simulink model "Copy_of_can_simple_block"  (Simulink 8.8)
settings: Solver=FixedStepDiscrete  StartTime=0.0  StopTime=1000  FixedStep=0.2  RelTol=1e-3  EnableMultiTasking=on
undefined symbols (not defined in the file or in its folder): A, A14, B, B13, B7, C, CS0, D, D4, F3, F4, G3, G4, H3, H4, K17, K4, L3, N16, N3, P3, PD4, PD5, PD6, R10, R14, SCK, SIN, SOUT, T14
libraries: rappid_564xl_ec_toolbox x16
settings Model: Creator=RMuradov  LastModifiedBy=User
settings DataIOCC: ExternalInput=off  InitialState=off  SaveOutput=off  SignalLogging=off  SaveTime=off
settings OptimizationCC: DefaultParameterBehavior=Inlined  ExpressionDepthLimit=2147483647  LifeSpan=1
settings DebuggingCC: SolverPrmCheckMsg=warning  InheritedTsInSrcMsg=none  SingleTaskRateTransMsg=error  UnconnectedInputMsg=error  UnconnectedOutputMsg=error  UnconnectedLineMsg=error  UnknownTsInhSupMsg=error
settings HardwareCC: ProdLargestAtomicInteger=Long  ProdLargestAtomicFloat=Double  ProdIntDivRoundTo=Zero  ProdEndianess=BigEndian  ProdHWDeviceType=Freescale->32-bit PowerPC
settings SFSimCC: SimCustomInitializer=init_PEC15_table();
settings SFSimCC: SimCustomHeaderCode=|
  | #include "doubleIt.h"
  | #include "PEC15.h"
settings SFSimCC: SimUserSources=|
  | doubleIt.c
  | PEC15.c
settings RTWCC: SystemTargetFile=rappid564xl.tlc  MakeCommand=rappid_564xl_make_rtw  TemplateMakefile=rappid_564xl_default_tmf  PostCodeGenCommand=rappid_analyzegencode(buildInfo)  Description=RAppID Toolbox MPC564xL Code Generation Target (rappid)  TLCAssert=on
settings CodeAppCC: IgnoreCustomStorageClasses=off  CustomSymbolStrType=$N$R$M  InternalIdentifier=Classic
settings STFCustomTargetCC: ModelReferenceCompliant=off  CombineOutputUpdateFcns=on  SuppressErrorStatus=on  ERTCustomFileBanners=on  SupportContinuousTime=off  SupportNonInlinedSFcns=off  RemoveResetFunc=on  MATLABClassNameForMDSCustomization=Simulink.SoftwareTarget.ERTCustomization  GRTInterface=off  SystemTargetFile=rappid564xl.tlc
settings ERTTargetCC: MultiwordLength=2048  ModelReferenceCompliant=off  ParMdlRefBuildCompliant=off  CompOptLevelCompliant=off  ConcurrentExecutionCompliant=off  SuppressErrorStatus=on  ERTFirstTimeCompliant=off  ModelStepFunctionPrototypeControlCompliant=off  CPPClassGenCompliant=off  UseToolchainInfoCompliant=off  ExtModeMexFile=noextcomm  InlinedParameterPlacement=NonHierarchical  ERTCustomFileTemplate=example_file_process.tlc  ConvertIfToSwitch=off  SuppressUnreachableDefaultCases=off

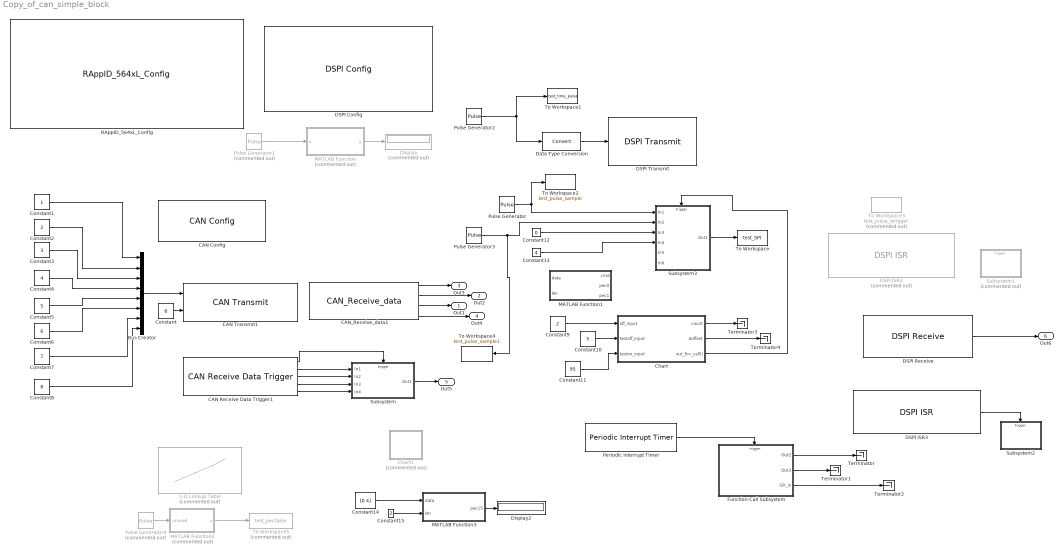
== system Copy_of_can_simple_block ==
  1-D Lookup Table : Lookup_n-D  Commented=on  NumberOfTableDimensions=1  BreakpointsForDimension1=[1:256]  Table="[0\t50585\t52907\t2866\t55503\t7510\t5732\t54269\t62471\t12702\t15020\t65333\t11464\t59729\t57955\t10234\t44439\t26638\t25404\t42661\t30040\t45249\t48115\t32362\t22928\t39945\t38715\t21154\t33119\t17606\t20468\t35437\t23342\t40631\t38277\t20508\t33761\t18040\t19786\t35027\t44841\t27312\t24962\t42011\t30694\t45695\t47437\t31956\t63161\t13088\t14354\t64907\t11894\t60399\t57565\t9540\t702\t50983\t52245\t2444\t55921\t8168\t5338\t53571\t62405\t13916\t15726\t63735\t11018\t61075\t58785\t8248\t1986\t49755\t51561\t3312\t57101\t6804\t4518\t54335\t24146\t39883\t37113\t21856\t34461\t17156\t18486\t36271\t43605\t28620\t25854\t41319\t29338\t46851\t48177\t31144\t43243\t28018\t26176\t41945\t28708\t46525\t48783\t31510\t23788\t39285\t37447\t22494\t33827\t16826\t19080\t36625\t1404\t49381\t52183\t3662\t56755\t6186\t4888\t54913\t61819\t13538\t16336\t64073\t10676\t60461\t59167\t8838\t41491\t26506\t27832\t43297\t31452\t48965\t46199\t29166\t22036\t37773\t39103\t23846\t36571\t19266\t16496\t34281\t3972\t51741\t49455\t1206\t55115\t4818\t6624\t56441\t64387\t15898\t13608\t61617\t9036\t59093\t60903\t10366\t63805\t15524\t14230\t61967\t8690\t58475\t61273\t10944\t3386\t51363\t50065\t1544\t54773\t4204\t7006\t57031\t21674\t37171\t39425\t24472\t35941\t18940\t17102\t34647\t41133\t25908\t28166\t43935\t30818\t48635\t46793\t29520\t20950\t37967\t40829\t23268\t35097\t19584\t18354\t33323\t42449\t24648\t27514\t44771\t32030\t47239\t46005\t30252\t64577\t14808\t13034\t63347\t9358\t57623\t59941\t12220\t2118\t52703\t50925\t884\t53385\t5392\t7714\t56251\t2808\t53089\t50259\t458\t53815\t6062\t7324\t55557\t65279\t15206\t12372\t62925\t9776\t58281\t59547\t11522\t42863\t25334\t27076\t44125\t32672\t47673\t45323\t29842\t21352\t38641\t40387\t22618\t35751\t20030\t17676\t32917]"  InternalRulePriority=Speed  RndMeth=Simplest  InputSameDT=on
  Bus Creator : BusCreator  Inputs=8
  CAN Config : rappid_564xl_ec_toolbox/MPC564xL/Communication Blocks/CAN Config  Priority=1  can_unit=A  can_unit_v2=0  can_idam=A - One full ID (standard or extended) per filter element.  can_srx_dis=1 - Self reception disabled  can_presdiv=4  can_rjw=3  can_pseg1=3  can_pseg2=3  can_clk_src=0 - The CAN engine clock source is the oscillator clock  can_lpb=0 - Loop Back disabled  can_smp=1 - Three samples are used to determine the value of the received bit  can_boff_rec=0 - Automatic recovering from Bus Off state enabled  can_tsyn=0 - Timer Sync feature disabled  can_lbuf=0 - Buffer with highest priority is transmitted first  can_lom=0 - Listen Only Mode is deactivated  can_propseg=6
  CAN Receive Data Trigger1 : rappid_564xl_ec_toolbox/MPC564xL/Communication Blocks/CAN Receive Data Trigger  can_unit=A  can_unit_v2=0  can_buffer=5  can_id=1021  can_isr_prio=14
  CAN Transmit1 : rappid_564xl_ec_toolbox/MPC564xL/Communication Blocks/CAN Transmit  can_unit=A  can_unit_v2=0  can_buffer=14  can_id=1020
  CAN_Receive_data1 : rappid_564xl_ec_toolbox/MPC564xL/Communication Blocks/CAN_Receive_data  can_unit=A  can_unit_v2=0  can_buffer=7  can_id=1010
  Chart : Stateflow chart  TreatAsAtomicUnit=on
  Chart1 : Stateflow chart  Commented=on  TreatAsAtomicUnit=on
  Constant : Constant  Value=8  OutDataTypeStr=uint8
  Constant1 : Constant  OutDataTypeStr=uint8
  Constant10 : Constant  Value=5
  Constant11 : Constant  Value=95
  Constant12 : Constant  Value=0  OutDataTypeStr=Inherit: Inherit via back propagation
  Constant13 : Constant  Value=4  OutDataTypeStr=Inherit: Inherit via back propagation
  Constant14 : Constant  Value=[0 4]  VectorParams1D=off  OutDataTypeStr=uint8
  Constant15 : Constant  Value=2  OutDataTypeStr=Inherit: Inherit via back propagation
  Constant2 : Constant  Value=2  OutDataTypeStr=uint8
  Constant3 : Constant  Value=3  OutDataTypeStr=uint8
  Constant4 : Constant  Value=4  OutDataTypeStr=uint8
  Constant5 : Constant  Value=5  OutDataTypeStr=uint8
  Constant6 : Constant  Value=6  OutDataTypeStr=uint8
  Constant7 : Constant  Value=7  OutDataTypeStr=uint8
  Constant8 : Constant  Value=8  OutDataTypeStr=uint8
  Constant9 : Constant  Value=2
  DSPI Config : rappid_564xl_ec_toolbox/MPC564xL/Communication Blocks/DSPI Config  Priority=1  dspi_Num=1  dspi_Mode=Master  dspi_MTFE=off  dspi_CONT_SCKE=off  dspi_PCSSE=off  dspi_ROOE=off  dspi_DIS_TXF=Enable  dspi_DIS_RXF_v2=Enable  dspi_SMPL_PT=DSPI samples SIN at driving SCK edge  dspi_FMSZ=16  dspi_CPOL=Low  dspi_CPHA=Data is captured on the leading edge of SCK and changed on the following edge  dspi_LSBFE=MSB first  dspi_DBR=off  dspi_PCSSCK=1  dspi_PASC=1  dspi_PDT=5  dspi_PBR=5  dspi_CSSCK=256  dspi_ASC=256  dspi_DT=8  dspi_BR=128  dspi_PCSIS0=High  dspi_PCSIS1=High  dspi_PCSIS2=High  dspi_PCSIS3=High  dspi_PCSIS4=High  dspi_PCSIS5=High  dspi_PCSIS6=High  dspi_PCSIS7=High  dspi_DIS_RXF=Oops
  DSPI ISR2 : rappid_564xl_ec_toolbox/MPC564xL/Communication Blocks/DSPI ISR  Commented=on  dspi_Num=1  dspi_isr_name=TCF - Transfer Complete  dspi_isrPrio=14  dspi_isr_tfuf=off  dspi_isr_rfof=on
  DSPI ISR3 : rappid_564xl_ec_toolbox/MPC564xL/Communication Blocks/DSPI ISR  dspi_Num=1  dspi_isr_name=EOQF - End of Queue  dspi_isrPrio=14  dspi_isr_tfuf=off  dspi_isr_rfof=on
  DSPI Receive : rappid_564xl_ec_toolbox/MPC564xL/Communication Blocks/DSPI Receive  dspi_Num=1
  DSPI Transmit : rappid_564xl_ec_toolbox/MPC564xL/Communication Blocks/DSPI Transmit  Priority=2  dspi_Num=1  dspi_CONT=off  dspi_PUSHR_PE=off  dspi_PUSHR_PP=off  dspi_PCS_0=36 : C[4] : [11] : [H3] : CS0  dspi_PCS_1=5 : A[5] : [14] : [H4] : CS0  dspi_PCS_2=3 : A[3] : [92] : [K17] : CS0  dspi_PCS_slave_0=36 : C[4] : [11] : [H3] : CS0  dspi_PCS_slave_1=5 : A[5] : [14] : [H4] : CS0  dspi_PCS_slave_2=3 : A[3] : [92] : [K17] : CS0  dspi_SIN_0=39 : C[7] : [15] : [K4] : SIN  dspi_SIN_1=8 : A[8] : [12] : [F4]  dspi_SIN_2=2 : A[2] : [84] : [N16] : SIN  dspi_SCK_0=37 : C[5] : [13] : [G3] : SCK  dspi_SCK_1=6 : A[6] : [2] : [G4] : SCK  dspi_SCK_2=0 : A[0] : [73] : [T14] : SCK  dspi_SOUT_0=38 : C[6] : [142] : [D4] : SOUT  dspi_SOUT_1=7 : A[7] : [10] : [F3] : SOUT  dspi_SOUT_2=1 : A[1] : [74] : [R14] : SOUT  dspi_Strobe=None  dspi_eoq=off  dspi_pcsx=Assert
  Data Type Conversion : DataTypeConversion  Priority=1
  Display : Display  Commented=on
  Display2 : Display
  Function-Call Subsystem : Subsystem  TreatAsAtomicUnit=on
      settings: RTWSystemCode=Nonreusable function
  MATLAB Function : MATLAB Function  Commented=on  TreatAsAtomicUnit=on
  MATLAB Function1 : MATLAB Function  TreatAsAtomicUnit=on
  MATLAB Function2 : MATLAB Function  Commented=on  TreatAsAtomicUnit=on
  MATLAB Function3 : MATLAB Function  TreatAsAtomicUnit=on
  Periodic Interrupt Timer : rappid_564xl_ec_toolbox/MPC564xL/General Purpose Blocks/Periodic Interrupt Timer  pit_chan=1  pit_timeout=200  int_priority=12  pit_timeout_val=23999999
  Pulse Generator : DiscretePulseGenerator  Period=100  PhaseDelay=3
  Pulse Generator1 : DiscretePulseGenerator  Commented=on  Amplitude=2  Period=100  PulseWidth=2
  Pulse Generator2 : DiscretePulseGenerator  Period=100
  Pulse Generator3 : DiscretePulseGenerator  Period=100  PhaseDelay=15
  Pulse Generator4 : DiscretePulseGenerator  Commented=on  Amplitude=2  Period=100  PulseWidth=2
  RAppID_564xL_Config : rappid_564xl_ec_toolbox/MPC564xL/RAppID_564xL_Config  SystemClock=120  XTAL=40  MC_clock_60=12  MC_clock_80=16  MC_clock_120=10  SWG_clock_60=20  SWG_clock_80=13.334  SWG_clock_120=20  Compiler=CodeWarrior  MemTarget=RAM  Part=MPC5643L  Package=144 LQFP  global_int_priority=11  base_tick_priority=12  sys_task_supress=off  exception_handlers=off  stored_mdl_name=can_simple_block__  freemaster_interface=Oops  freemaster_rx_pin="LINFlex_0 Rx Pin 116 : \"PB[3]\""  freemaster_tx_pin="LINFlex_0 Tx Pin 114 : \"PB[2]\""  freemaster_interface_1=None  freemaster_enable=off  freemaster_rate=57600  freemaster_tx0_pin=18 : B[2] : 114 : A14  freemaster_rx0_pin=19 : B[3] : 116 : B13  freemaster_tx1_pin=57 : D[9] : 26 : L3  freemaster_rx1_pin=29 : B[13] : 60 : R10  freemaster_can_channel=1CH  freemater_can_speed=500K  freemaster_can_msgig=0x7AA  ccp_interface=None  ccp_enable=off  ccp_can_channel=CH1 (MB 0 - 1)  ccp_can_speed=500K  ccp_can_cro_id=256  ccp_can_dto_id=257  ccp_dev_id=RappID  ccp_dev_addr=0  ccp_odt=3  ccp_daq=3  pil_enable=off  pil_bam=off  comport=1  pil_rate=57600  bam_password_def=on  bam_password=0xFEEDFACECAFEBEEF  bam_sa_cs=off  bam_start_address=0x0  bam_code_size=0x7000  cons_dspi=on  cons_can=on  cons_adc=on  cons_pwm=on  cons_ctu=on  cons_swg=on  cons_eTimer=on  cons_fm=on
  Subsystem : Subsystem
      settings: RTWSystemCode=Nonreusable function
  Subsystem1 : Subsystem  Commented=on
      settings: RTWSystemCode=Nonreusable function
  Subsystem2 : Subsystem
      settings: RTWSystemCode=Nonreusable function
  Subsystem3 : Subsystem
      settings: RTWSystemCode=Nonreusable function
  Terminator{,1..4} (5 alike) : Terminator
  To Workspace : ToWorkspace  VariableName=test_SPI  SaveFormat=Timeseries  SampleTime=-1
  To Workspace1 : ToWorkspace  VariableName=test_time_pulse  SaveFormat=Timeseries  SampleTime=-1
  To Workspace2 : ToWorkspace  VariableName=test_pulse_sample  SaveFormat=Timeseries  SampleTime=-1
  To Workspace3 : ToWorkspace  Commented=on  VariableName=test_pulse_strigger  SaveFormat=Timeseries  SampleTime=-1
  To Workspace4 : ToWorkspace  VariableName=test_pulse_sample1  SaveFormat=Timeseries  SampleTime=-1
  To Workspace5 : ToWorkspace  Commented=on  VariableName=test_pectable  SampleTime=-1
      settings: Save2DSignal=2-D array (concatenate along first dimension)
  Out1 : Outport
  Out2 : Outport  Port=2
  Out3 : Outport  Port=3
  Out4 : Outport  Port=4
  Out5 : Outport  Port=5
  Out6 : Outport  Port=6
  wires:
  Bus Creator/1 -> CAN Transmit1/1
  Constant1/1 -> Bus Creator/1
  Constant2/1 -> Bus Creator/2
  Constant3/1 -> Bus Creator/3
  Constant4/1 -> Bus Creator/4
  Constant5/1 -> Bus Creator/5
  Constant6/1 -> Bus Creator/6
  Constant8/1 -> Bus Creator/8
  Constant7/1 -> Bus Creator/7
  CAN_Receive_data1/4 -> Out4/1
  CAN_Receive_data1/3 -> Out1/1
  CAN_Receive_data1/2 -> Out2/1
  CAN_Receive_data1/1 -> Out3/1
  Constant/1 -> CAN Transmit1/2
  CAN Receive Data Trigger1/3 -> Subsystem/2(In2)
  CAN Receive Data Trigger1/4 -> Subsystem/3(In3)
  CAN Receive Data Trigger1/5 -> Subsystem/4(In4)
  CAN Receive Data Trigger1/2 -> Subsystem/1(In1)
  CAN Receive Data Trigger1/1 -> Subsystem/Trigger
  Subsystem/1(Out1) -> Out5/1
  DSPI Receive/1 -> Out6/1
  DSPI ISR3/1 -> Subsystem2/Trigger
  Data Type Conversion/1 -> DSPI Transmit/1
  Periodic Interrupt Timer/1 -> Function-Call Subsystem/Trigger
  Function-Call Subsystem/1(Out2) -> Terminator/1
  Function-Call Subsystem/2(Out3) -> Terminator1/1
  Function-Call Subsystem/3(SPI_in) -> Terminator2/1
  Pulse Generator/1 -> Subsystem3/1(In1), To Workspace2/1
  Subsystem3/1(Out1) -> To Workspace/1
  Pulse Generator1/1 -> MATLAB Function/1(u)
  MATLAB Function/1(y) -> Display/1
  Pulse Generator2/1 -> Data Type Conversion/1, To Workspace1/1
  Chart/1(count) -> Terminator3/1
  Chart/2(" Aoffset") -> Terminator4/1
  Chart/3(out_fcn_call()) -> Subsystem3/Trigger
  Pulse Generator3/1 -> Subsystem3/2(In2), To Workspace4/1
  Constant9/1 -> Chart/1(off_input)
  Constant10/1 -> Chart/2(testoff_input)
  Constant11/1 -> Chart/3(teston_input)
  MATLAB Function2/1(y) -> To Workspace5/1
  Pulse Generator4/1 -> MATLAB Function2/1(unused)
  Constant14/1 -> MATLAB Function3/1(data)
  Constant15/1 -> MATLAB Function3/2(len)
  MATLAB Function3/1(pec15) -> Display2/1
  Constant12/1 -> Subsystem3/3(In3)
  Constant13/1 -> Subsystem3/4(In4)

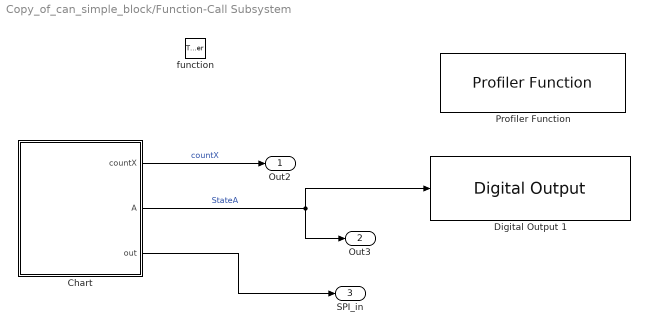
== system Copy_of_can_simple_block/Function-Call Subsystem ==
  function : TriggerPort  TriggerType=function-call  VariantControl=Variant
  Chart : Stateflow chart  TreatAsAtomicUnit=on
  Digital Output 1 : rappid_564xl_ec_toolbox/MPC564xL/General Purpose Blocks/Digital Output   gpio_outputs="52  : PD4  : [ 129 ] : [ B7 ]"  pinNum=[ 129 ]  pcrNum=52
  "Profiler Function " : rappid_564xl_ec_toolbox/MPC564xL/Utility Blocks/Profiler Function   profile_indx=0
  Out2 : Outport
  Out3 : Outport  Port=2
  SPI_in : Outport  Port=3
  wires:
  Chart/1(countX) -> Out2/1  "countX"
  Chart/2(" A") -> Out3/1, Digital Output 1/1  "StateA"
  Chart/3(out) -> SPI_in/1

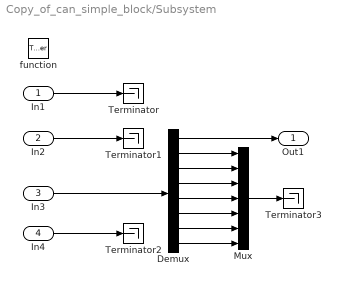
== system Copy_of_can_simple_block/Subsystem ==
  In1 : Inport
  In2 : Inport  Port=2
  In3 : Inport  Port=3
  In4 : Inport  Port=4
  function : TriggerPort  TriggerType=function-call  VariantControl=Variant
  Demux : Demux  Outputs=8
  Mux : Mux  Inputs=7
  Terminator{,1..3} (4 alike) : Terminator
  Out1 : Outport
  wires:
  In1/1 -> Terminator/1
  In2/1 -> Terminator1/1
  In4/1 -> Terminator2/1
  In3/1 -> Demux/1
  Demux/8 -> Mux/7
  Demux/7 -> Mux/6
  Demux/6 -> Mux/5
  Demux/5 -> Mux/4
  Demux/4 -> Mux/3
  Demux/3 -> Mux/2
  Demux/2 -> Mux/1
  Mux/1 -> Terminator3/1
  Demux/1 -> Out1/1

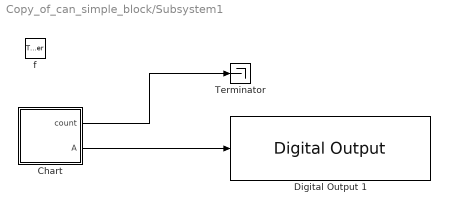
== system Copy_of_can_simple_block/Subsystem1 ==
  f : TriggerPort  TriggerType=function-call  VariantControl=Variant
  Chart : Stateflow chart  TreatAsAtomicUnit=on
  Digital Output 1 : rappid_564xl_ec_toolbox/MPC564xL/General Purpose Blocks/Digital Output   gpio_outputs="53  : PD5  : [ 33 ] : [ N3 ]"  pinNum=[ 33 ]  pcrNum=53
  Terminator : Terminator
  wires:
  Chart/1(count) -> Terminator/1
  Chart/2(" A") -> Digital Output 1/1

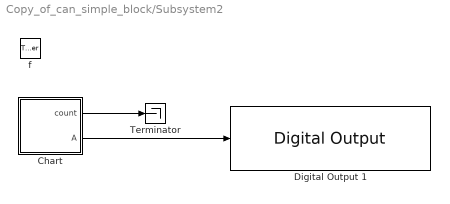
== system Copy_of_can_simple_block/Subsystem2 ==
  f : TriggerPort  TriggerType=function-call  VariantControl=Variant
  Chart : Stateflow chart  TreatAsAtomicUnit=on
  Digital Output 1 : rappid_564xl_ec_toolbox/MPC564xL/General Purpose Blocks/Digital Output   gpio_outputs="54  : PD6  : [ 34 ] : [ P3 ]"  pinNum=[ 34 ]  pcrNum=54
  Terminator : Terminator
  wires:
  Chart/1(count) -> Terminator/1
  Chart/2(" A") -> Digital Output 1/1

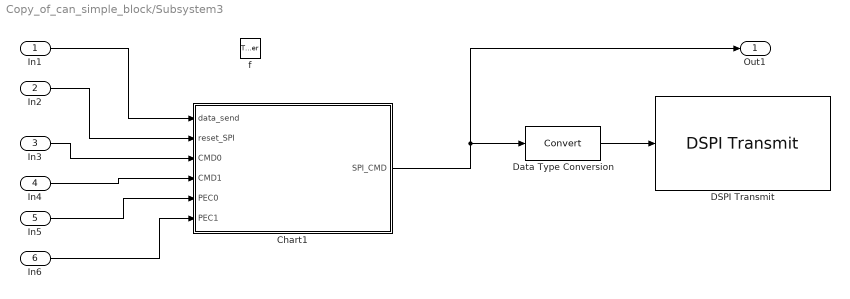
== system Copy_of_can_simple_block/Subsystem3 ==
  In1 : Inport
  In2 : Inport  Port=2
  In3 : Inport  Port=3
  In4 : Inport  Port=4
  In5 : Inport  Port=5
  In6 : Inport  Port=6
  f : TriggerPort  TriggerType=function-call  VariantControl=Variant
  Chart1 : Stateflow chart  TreatAsAtomicUnit=on
  DSPI Transmit : rappid_564xl_ec_toolbox/MPC564xL/Communication Blocks/DSPI Transmit  Priority=2  dspi_Num=1  dspi_CONT=off  dspi_PUSHR_PE=off  dspi_PUSHR_PP=off  dspi_PCS_0=36 : C[4] : [11] : [H3] : CS0  dspi_PCS_1=5 : A[5] : [14] : [H4] : CS0  dspi_PCS_2=3 : A[3] : [92] : [K17] : CS0  dspi_PCS_slave_0=36 : C[4] : [11] : [H3] : CS0  dspi_PCS_slave_1=5 : A[5] : [14] : [H4] : CS0  dspi_PCS_slave_2=3 : A[3] : [92] : [K17] : CS0  dspi_SIN_0=39 : C[7] : [15] : [K4] : SIN  dspi_SIN_1=8 : A[8] : [12] : [F4]  dspi_SIN_2=2 : A[2] : [84] : [N16] : SIN  dspi_SCK_0=37 : C[5] : [13] : [G3] : SCK  dspi_SCK_1=6 : A[6] : [2] : [G4] : SCK  dspi_SCK_2=0 : A[0] : [73] : [T14] : SCK  dspi_SOUT_0=38 : C[6] : [142] : [D4] : SOUT  dspi_SOUT_1=7 : A[7] : [10] : [F3] : SOUT  dspi_SOUT_2=1 : A[1] : [74] : [R14] : SOUT  dspi_Strobe=None  dspi_eoq=off  dspi_pcsx=Assert
  Data Type Conversion : DataTypeConversion  Priority=1
  Out1 : Outport
  wires:
  Chart1/1(SPI_CMD) -> Data Type Conversion/1, Out1/1
  In1/1 -> Chart1/1(data_send)
  Data Type Conversion/1 -> DSPI Transmit/1
  In2/1 -> Chart1/2(reset_SPI)
  In3/1 -> Chart1/3(CMD0)
  In4/1 -> Chart1/4(CMD1)
  In5/1 -> Chart1/5(PEC0)
  In6/1 -> Chart1/6(PEC1)

== stateflow chart Subsystem2/Chart ==
  state A
  state A1
  (default) -> A : {count =0;}
  A -> A1
  A1 -> A : { count = count + 1;}
  data: count output double; A output boolean

== stateflow chart Function-Call Subsystem/Chart ==
  state A
    entry: out=0;
    du: out=0;
  state A1
    entry: out=1;
    du: out=1;
  state A2
    entry: out=2;
    du: out=2;
  (default) -> A
  A2 -> A : { countX = countX + 0.01;}
  A -> A1
  A1 -> A2
  data: countX output single [0..10000]; A output boolean [0..1]; out output double

== stateflow chart Subsystem3/Chart1 ==
  state State0
    en:SPI_CMD=CMD(i);
    du:SPI_CMD = CMD(i);
  state State2
    en:SPI_CMD=CMD1;
    du:SPI_CMD = CMD1;
  state State3
    en:SPI_CMD=PEC0;
    du:SPI_CMD = PEC0;
  state State4
    en:SPI_CMD=PEC1;
    du:SPI_CMD = PEC1;
  state State5
    en:SPI_CMD=6;
    du:SPI_CMD = 6;
  (default) -> State0
  State5 -> State0
  State0 -> State2 : [data_send == 1]
  State3 -> State0 [order 2] : [reset_SPI == 1]
  State4 -> State0 [order 2] : [reset_SPI == 1]
  State2 -> State3
  State4 -> State5 [order 1] : [reset_SPI ~= 1]
  State3 -> State4 [order 1] : [reset_SPI ~= 1]
  data: SPI_CMD output double; data_send input double; reset_SPI input double; CMD0 input uint8; CMD1 input uint8; PEC0 input uint8; PEC1 input uint8

== matlab function MATLAB Function ==
  data: u input double; y output uint16
function y = callingDoubleIt(u)

y = 0.0;
y = coder.ceval('doubleIt',u);

== stateflow chart Subsystem1/Chart ==
  state A
  state A1
  (default) -> A : {count =0;}
  A -> A1
  A1 -> A : { count = count + 1;}
  data: count output double; A output boolean

== stateflow chart Chart ==
  state Aoffset
    en:offcnt = 1;
    du:offcnt = offcnt + 1;
  state Aon
    en:testoncnt=1;
    du:testoncnt=testoncnt+1;
    du:out_fcn_call;
  state Aoff
    en:testoffcnt=1;
    du:testoffcnt=testoffcnt+1;
  (default) -> Aoffset : {count =0;}
  Aoffset -> Aon : [offcnt >= off_input]
  Aoff -> Aon : [testoffcnt >= testoff_input]
  Aon -> Aoff : [testoncnt >= teston_input]
  data: count output double; Aoffset output boolean; testcnt local double; off_input input double; testoff_input input double; teston_input input double; offcnt local double; testoffcnt local double; testoncnt local double
  events: out_fcn_call output FUNCTION_CALL_EVENT

== stateflow chart Chart1 ==
  state INIT
  state SLEEP
  state STANDBY
  state WAIT
  state DATA_RECEIVE
  state CONFIG
  state CONFIG_WAIT
  (default) -> INIT
  INIT -> CONFIG
  CONFIG -> CONFIG_WAIT
  CONFIG_WAIT -> STANDBY
  SLEEP -> STANDBY
  STANDBY -> SLEEP [order 2]
  DATA_RECEIVE -> STANDBY
  STANDBY -> WAIT [order 1]
  WAIT -> DATA_RECEIVE

== matlab function MATLAB Function2 ==
  data: unused input double; y output uint16
function y  = initPecTable(~)

yy = uint16(zeros(1,256));
remaindertest = uint16(zeros(1,256));
d = uint16(hex2dec('4000'));
CRC15_POLY = uint16(hex2dec('4599'));
onemask16 = uint16(hex2dec('FFFF'));

for i=0:255
    ii = uint16(i);
    remainder = uint16(bitshift(ii,7));
    for bit=8:-1:1
        if (bitand(remainder,d,'uint16') ~= 0)
            remainder = uint16(bitshift(remainder,1));
            remainder = uint16(bitxor(remainder,CRC15_POLY,'uint16'));
        else
            remainder = uint16(bitshift(remainder,1));            
        end
    end
    remaindertest(1,ii+1) = remainder;
    yy(1,ii+1) = uint16(bitand(remainder,onemask16,'uint16'));
end
y = yy;

== matlab function MATLAB Function3 ==
  data: data input double; len input double; pec15 output double
function pec15  = fcn(data,len)

data_uint8 = uint8(data);
pec15Table = [0 50585 52907 2866 55503 7510 5732 54269 62471 12702 15020 65333 ...
    11464 59729 57955 10234 44439	26638	25404	42661	30040	45249	48115	32362	22928	39945	38715	21154	33119	17606	20468	35437	23342	40631	38277	20508	33761	18040	19786	35027	44841	27312	24962	42011	30694	45695	47437	31956	63161	13088	14354	64907	11894	60399	57565	9540	702	50983	52245	2444	55921	8168	5338	53571	62405	13916	15726	63735	11018	61075	58785	8248	1986	49755	51561	3312	57101	6804	4518	54335	24146	39883	37113	21856	34461	17156	18486	36271	43605	28620	25854	41319	29338	46851	48177	31144	43243	28018	26176	41945	28708	46525	48783	31510	23788	39285	37447	22494	33827	16826	19080	36625	1404	49381	52183	3662	56755	6186	4888	54913	61819	13538	16336	64073	10676	60461	59167	8838	41491	26506	27832	43297	31452	48965	46199	29166	22036	37773	39103	23846	36571	19266	16496	34281	3972	51741	49455	1206	55115	4818	6624	56441	64387	15898	13608	61617	9036	59093	60903	10366	63805	15524	14230	61967	8690	58475	61273	10944	3386	51363	50065	1544	54773	4204	7006	57031	21674	37171	39425	24472	35941	18940	17102	34647	41133	25908	28166	43935	30818	48635	46793	29520	20950	37967	40829	23268	35097	19584	18354	33323	42449	24648	27514	44771	32030	47239	46005	30252	64577	14808	13034	63347	9358	57623	59941	12220	2118	52703	50925	884	53385	5392	7714	56251	2808	53089	50259	458	53815	6062	7324	55557	65279	15206	12372	62925	9776	58281	59547	11522	42863	25334	27076	44125	32672	47673	45323	29842	21352	38641	40387	22618	35751	20030	17676	32917];
onemask8 = uint8(hex2dec('FF'));
onemask16 = uint16(hex2dec('FFFF'));

% data_test = zeros(1,2);
remainder = uint16(16);

for i=1:len
    ii = uint16(i);
%     data_test(1,i) = data(ii); 
%     address = 2;
    address = bitand( ...
        bitxor( ...
        uint8(bitsra(remainder,7)),data(ii) ), ...
        onemask8);
    remainder = bitxor(bitshift(remainder,8,'uint16'),pec15Table(address+1));
end
pec15 = uint16(bitand(bitshift(remainder,1,'uint16'),onemask16));




% int pec15(char data[], int len){
%     int remainder, address, i;
%     remainder = 16;
%     for (i=0;i<len;i++){
%         address = ((remainder >> 7)^data[i])&0xFF;
%         remainder = (remainder << 8) ^ pec15Table[address];
%     }
%     return (remainder*2);
% }

== matlab function MATLAB Function1 ==
  data: data input double; len input double; cmd output double; pec0 output double; pec1 output double
function [cmd, pec0, pec1]  = fcn(data,len)

data_uint8 = uint8(data);
pec15Table = [0 50585 52907 2866 55503 7510 5732 54269 62471 12702 15020 65333 ...
    11464 59729 57955 10234 44439 26638 25404 42661 30040 45249 48115 ... 
    32362 22928 39945 38715	21154	33119	17606	20468	35437	23342	40631	38277	20508	33761	18040	19786	35027	44841	27312	24962	42011	30694	45695	47437	31956	63161	13088	14354	64907	11894	60399	57565	9540	702	50983	52245	2444	55921	8168	5338	53571	62405	13916	15726	63735	11018	61075	58785	8248	1986	49755	51561	3312	57101	6804	4518	54335	24146	39883	37113	21856	34461	17156	18486	36271	43605	28620	25854	41319	29338	46851	48177	31144	43243	28018	26176	41945	28708	46525	48783	31510	23788	39285	37447	22494	33827	16826	19080	36625	1404	49381	52183	3662	56755	6186	4888	54913	61819	13538	16336	64073	10676	60461	59167	8838	41491	26506	27832	43297	31452	48965	46199	29166	22036	37773	39103	23846	36571	19266	16496	34281	3972	51741	49455	1206	55115	4818	6624	56441	64387	15898	13608	61617	9036	59093	60903	10366	63805	15524	14230	61967	8690	58475	61273	10944	3386	51363	50065	1544	54773	4204	7006	57031	21674	37171	39425	24472	35941	18940	17102	34647	41133	25908	28166	43935	30818	48635	46793	29520	20950	37967	40829	23268	35097	19584	18354	33323	42449	24648	27514	44771	32030	47239	46005	30252	64577	14808	13034	63347	9358	57623	59941	12220	2118	52703	50925	884	53385	5392	7714	56251	2808	53089	50259	458	53815	6062	7324	55557	65279	15206	12372	62925	9776	58281	59547	11522	42863	25334	27076	44125	32672	47673	45323	29842	21352	38641	40387	22618	35751	20030	17676	32917];
onemask8 = uint8(hex2dec('FF'));
onemask8_8sft = uint8(hex2dec('FF00'));
onemask16 = uint16(hex2dec('FFFF'));

% data_test = zeros(1,2);
remainder = uint16(16);

for i=1:len
    ii = uint16(i);
%     data_test(1,i) = data(ii); 
%     address = 2;
    address = bitand( ...
        bitxor( ...
        uint8(bitsra(remainder,7)),data(ii) ), ...
        onemask8);
    remainder = bitxor(bitshift(remainder,8,'uint16'),pec15Table(address+1));
end
pec15 = uint16(bitand(bitshift(remainder,1,'uint16'),onemask16));
pec0 = uint8(bitand(pec15,onemask8));
pec1 = uint8(bitsra(bitand(pec15,onemask8_8sft)),8);




% int pec15(char data[], int len){
%     int remainder, address, i;
%     remainder = 16;
%     for (i=0;i<len;i++){
%         address = ((remainder >> 7)^data[i])&0xFF;
%         remainder = (remainder << 8) ^ pec15Table[address];
%     }
%     return (remainder*2);
% }
